simulink model "benchlink"  (R2024b)
settings: Solver=FixedStepDiscrete  StartTime=0.0  StopTime=0.005*16  RelTol=1e-3
model workspace (MAT data in the model file):
  socvcb : containers.Map (value not decoded)
values from neighbouring files (symbols this model uses):
  access = [32 0 4 36 32 0 4 36 32 0 4 36 ... (16 elements, 16x1)]    [all_variables.mat]
  qam_params =     [all_variables.mat]
undefined symbols (not defined in the file or in its folder): Add, j, QAM, rms, Shift
libraries: hdlsllib x53, simulink_need_slupdate x22, simulink x18, dspsigops x16, commdigbbndam3 x6, dsphdlmathfun2 x2, commchan3 x1, commrflib2 x1, dsphdlsigops2 x1, dspstat3 x1, dsphdlfiltering2 x1, simulink_extras x1
(part 4 of 5)

== system benchlink/HDL_64QAM/HDLRxIPCore/QAM Rx HDL/MF Filtering and Despreading/SymEVM ==
  chipValid : Inport
  chips : Inport  Port=2
  switchControl : Inport  Port=3
  " Integrate and Dump" : MATLAB Function  TreatAsAtomicUnit=on
  Add2 : Sum  Inputs=-+  OutDataTypeStr=fixdt(1,16,11)  SaturateOnIntegerOverflow=on
  Constant1 : Constant  Value=complex(0,0)  OutDataTypeStr=fixdt(1,32,15)  SampleTime=1/qam_params.chipRate
  Data Type Conversion3 : DataTypeConversion  OutDataTypeStr=fixdt(1,16,14)  RndMeth=Floor
  Delay{1..3,5..9,11..13,15,20..21} (14 alike) : Delay  DelayLength=1  InitialCondition=0  UseCircularBuffer=on
  Delay14 : Delay  DelayLength=9  InitialCondition=0  UseCircularBuffer=on
  Delay4 : Delay  Commented=on  DelayLength=1  InitialCondition=0  UseCircularBuffer=on
  Modulus : Subsystem
  Rectangular QAM Demodulator Baseband1 : commdigbbndam3/Rectangular QAM Demodulator Baseband  M=64  OutType=Integer  DecType=Hard decision  VarSource=Dialog  Variance=1  Dec=Gray  Mapping=[0:15]  PowType=Min. distance between symbols  MinDist=2  AvgPow=0.66  PeakPow=1  Ph=0  outDtype1=boolean  outDtype2=Inherit via internal rule  derotateFactorWordLen=16  derotateFactorDataTypeStr=Inherit: Same word length as input  derotateFactorLastDataTypeStr=Inherit: Same word length as input  denormFactorWordLen=16  denormFactorDataTypeStr=Inherit: Same word length as input  denormFactorLastDataTypeStr=Inherit: Same word length as input  prodOutWordLen=32  prodOutOverflowMode=Wrap  prodOutRoundingMode=Floor  prodOutOvFlMode=off  prodOutOvFlModeLastStrValue=off  sumWordLen=32
  Rectangular QAM Modulator Baseband1 : commdigbbndam3/Rectangular QAM Modulator Baseband  M=64  InType=Integer  Enc=Gray  Mapping=[0:15]  PowType=Min. distance between symbols  MinDist=2  AvgPow=.66  PeakPow=1.1  Ph=0  outDtype=Fixed-point  outWordLen=16  outUDDataType=sfix(16)  outFracLenMode=Best precision  outFracLen=15  outDataTypeStr=fixdt(1,16)  outLastDataTypeStr=fixdt(1,16)
  SEL2 : MultiPortSwitch  DataPortOrder=Zero-based contiguous  Inputs=2  DiagnosticForDefault=None  zeroidx=on  OutDataTypeStr=fixdt(1,32,15)  InputSameDT=off
  Shift Arithmetic1 : ArithShift  BinPtShiftNumber=-3  BitShiftDirection=Right
  Shift Arithmetic2 : ArithShift  BinPtShiftNumber=3  BitShiftDirection=Right
  Symbol Accum : Subsystem
  Unit Delay Enabled1 : simulink_need_slupdate/Unit Delay Enabled  vinit=0.0  tsamp=-1
  EVM : Outport  InitialOutput=0  VectorParamsAs1DForOutWhenUnconnected=off
  wires:
  chips/1 -> Delay13/1
  Delay21/1 -> Delay1/1
  Delay20/1 -> Data Type Conversion3/1
  " Integrate and Dump"/2(sumOut) -> Delay20/1
  " Integrate and Dump"/1(validOut) -> Delay21/1
  Delay13/1 -> " Integrate and Dump"/2(symbolIn)
  Symbol Accum/2(ValidOut) -> Unit Delay Enabled1/2
  Symbol Accum/1(Out) -> Unit Delay Enabled1/1
  Delay14/1 -> Symbol Accum/1(SwCtrl)
  Delay11/1 -> Delay12/1
  Data Type Conversion3/1 -> Shift Arithmetic2/1
  Modulus/1(dataOut) -> Delay15/1
  Unit Delay Enabled1/1 -> EVM/1
  Add2/1 -> Shift Arithmetic1/1  "e"
  Rectangular QAM Modulator Baseband1/1 -> Delay7/1
  Delay6/1 -> Rectangular QAM Demodulator Baseband1/1
  Delay12/1 -> Delay8/1
  Delay15/1 -> Symbol Accum/2(In)
  Delay9/1 -> Rectangular QAM Modulator Baseband1/1
  Rectangular QAM Demodulator Baseband1/1 -> Delay9/1
  Constant1/1 -> SEL2/2
  SEL2/1 -> Add2/1
  Delay1/1 -> Delay2/1
  Delay2/1 -> Delay5/1
  chipValid/1 -> Delay3/1
  Delay3/1 -> [chipValid], " Integrate and Dump"/1(dValid)
  [chipValid] -> Delay14/1
  Shift Arithmetic2/1 -> Delay6/1, Delay11/1
  Shift Arithmetic1/1 -> Modulus/1(dataIn)
  Delay8/1 -> Add2/2
  Delay7/1 -> SEL2/3
  Delay5/1 -> SEL2/1
  switchControl/1 -> Symbol Accum/3(switchControl)

== system benchlink/HDL_64QAM/HDLRxIPCore/QAM Rx HDL/Payload Delimiter/Normalized Modulus ==
  dataIn : Inport
  switchControl : Inport  Port=2
  Abs : Abs
  Abs1 : Abs
  Add : Sum  OutDataTypeStr=fixdt(0,8,8)  SaturateOnIntegerOverflow=on
  Add7 : Sum  SaturateOnIntegerOverflow=on
  Complex to Real-Imag2 : ComplexToRealImag
  Constant1 : Constant  Value=2^(-14)  OutDataTypeStr=fixdt(0,16,14)  SampleTime=-1
  Delay{1..9,15..16} (11 alike) : Delay  DelayLength=1  InitialCondition=0
  Delay10 : Delay  DelayLength=length(PreAmb)  InitialCondition=0
  Gain4 : Gain  Gain=0.4  OutDataTypeStr=fixdt(1,16,15)  SaturateOnIntegerOverflow=on
  KeepMax : MATLAB Function  TreatAsAtomicUnit=on
  KeepMaxSmallBurst : MATLAB Function  TreatAsAtomicUnit=on
  MinMax : MinMax  Inputs=2  SaturateOnIntegerOverflow=on
  MinMax1 : MinMax  Function=max  Inputs=2  SaturateOnIntegerOverflow=on
  Multiport Switch : MultiPortSwitch  Inputs=2  SaturateOnIntegerOverflow=off  InputSameDT=off
  Product : Product  SaturateOnIntegerOverflow=on
  Reciprocal : Product  Inputs=/  OutDataTypeStr=fixdt(0,8,1)  RndMeth=Zero  SaturateOnIntegerOverflow=on
  dataOut : Outport  VectorParamsAs1DForOutWhenUnconnected=off
  dataOutN : Outport  Port=2  VectorParamsAs1DForOutWhenUnconnected=off
  wires:
  dataIn/1 -> Complex to Real-Imag2/1
  Abs1/1 -> Delay1/1
  Abs/1 -> Delay4/1
  Gain4/1 -> Delay6/1
  MinMax1/1 -> Delay2/1  "|L|"
  MinMax/1 -> Delay7/1  "|Q|"
  Add7/1 -> Delay5/1
  Delay7/1 -> Gain4/1
  Delay2/1 -> Delay3/1
  Delay1/1 -> MinMax1/2, MinMax/2
  Delay4/1 -> MinMax1/1, MinMax/1
  Delay6/1 -> Add7/2
  Delay3/1 -> Add7/1
  Complex to Real-Imag2/2 -> Abs1/1  "Q"
  Complex to Real-Imag2/1 -> Abs/1  "I"
  Delay15/1 -> Add/1
  Add/1 -> Reciprocal/1
  Constant1/1 -> Add/2
  Product/1 -> Delay16/1
  KeepMax/1(out) -> Multiport Switch/2
  Delay16/1 -> dataOutN/1
  Delay8/1 -> Product/1, Delay9/1
  Delay9/1 -> dataOut/1
  Delay5/1 -> Delay10/1, KeepMaxSmallBurst/1(in), KeepMax/1(in)
  Delay10/1 -> Delay8/1
  Reciprocal/1 -> Product/2
  switchControl/1 -> Multiport Switch/1
  KeepMaxSmallBurst/1(out) -> Multiport Switch/3
  Multiport Switch/1 -> Delay15/1

== system benchlink/HDL_64QAM/HDLRxIPCore/QAM Rx HDL/Payload Delimiter/Peak Detector ==
  xCorr : Inport
  Threshold : Inport  Port=2
  Compare To Zero : simulink/Logic and Bit Operations/Compare To Zero  relop=>  OutDataTypeStr=boolean
  Compare To Zero1 : simulink/Logic and Bit Operations/Compare To Zero  relop=>  OutDataTypeStr=boolean
  Delay : Delay  DelayLength=1
  Delay1 : Delay
  Delay4 : Delay  DelayLength=1
  Logical Operator1 : Logic  AllPortsSameDT=off  OutDataTypeStr=boolean
  Logical Operator3 : Logic  AllPortsSameDT=off  OutDataTypeStr=boolean
  Subtract1 : Sum  Inputs=-+
  Subtract2 : Sum  Inputs=+-
  Out1 : Outport  VectorParamsAs1DForOutWhenUnconnected=off
  wires:
  Threshold/1 -> Delay4/1
  Delay/1 -> Subtract1/2, Subtract2/1
  Delay1/1 -> Subtract2/2
  xCorr/1 -> Delay1/1, Subtract1/1, Delay/1
  Delay4/1 -> Logical Operator3/1
  Subtract1/1 -> Compare To Zero/1
  Subtract2/1 -> Compare To Zero1/1
  Compare To Zero/1 -> Logical Operator1/1
  Compare To Zero1/1 -> Logical Operator1/2
  Logical Operator1/1 -> Logical Operator3/2
  Logical Operator3/1 -> Out1/1

== system benchlink/HDL_64QAM/HDLRxIPCore/QAM Rx HDL/Payload Delimiter/Preamble Matched Filter ==
  dataIn : Inport
  Add2 : Sum  SaturateOnIntegerOverflow=on
  Add3 : Sum  SaturateOnIntegerOverflow=on
  Complex to Real-Imag2 : ComplexToRealImag
  Delay{1,4..6} (4 alike) : Delay  DelayLength=1  InitialCondition=0
  Discrete FIR Filter1 : DiscreteFir  FilterStructure=Direct form transposed  Coefficients=sign(real(fliplr(PreAmb)))  CoefDataTypeStr=fixdt(1,2,0)  ProductDataTypeStr=fixdt(1,16,15)  AccumDataTypeStr=fixdt(1,24,15)  OutDataTypeStr=fixdt(1,24,15)  SaturateOnIntegerOverflow=on
  Discrete FIR Filter2 : DiscreteFir  FilterStructure=Direct form transposed  Coefficients=sign(imag(fliplr(PreAmb)))  CoefDataTypeStr=fixdt(1,2,0)  ProductDataTypeStr=fixdt(1,16,15)  AccumDataTypeStr=fixdt(1,24,15)  OutDataTypeStr=fixdt(1,24,15)  SaturateOnIntegerOverflow=on
  Gain : Gain  Gain=1/length(PreAmb)  OutDataTypeStr=fixdt(1,17,15)  SaturateOnIntegerOverflow=on
  Gain1 : Gain  Gain=1/length(PreAmb)  OutDataTypeStr=fixdt(1,17,15)  SaturateOnIntegerOverflow=on
  Real-Imag to Complex1 : RealImagToComplex
  dataOut : Outport  VectorParamsAs1DForOutWhenUnconnected=off
  wires:
  Delay1/1 -> Discrete FIR Filter2/1
  Delay4/1 -> Discrete FIR Filter1/1
  Add3/1 -> Delay1/1
  Add2/1 -> Delay4/1
  Complex to Real-Imag2/1 -> Add3/1, Add2/1
  Complex to Real-Imag2/2 -> Add2/2, Add3/2
  dataIn/1 -> Complex to Real-Imag2/1
  Delay5/1 -> Real-Imag to Complex1/1
  Delay6/1 -> Real-Imag to Complex1/2
  Gain/1 -> Delay5/1
  Discrete FIR Filter1/1 -> Gain/1
  Discrete FIR Filter2/1 -> Gain1/1
  Gain1/1 -> Delay6/1
  Real-Imag to Complex1/1 -> dataOut/1

== system benchlink/HDL_64QAM/HDLRxIPCore/QAM Rx HDL/Payload Delimiter/Rising Edge Detector ==
  In1 : Inport
  Compare To Constant7 : simulink/Logic and Bit Operations/Compare To Constant  relop===  const=1  OutDataTypeStr=boolean
  Data Type Conversion : DataTypeConversion  OutDataTypeStr=fixdt(1,2,0)  SaturateOnIntegerOverflow=off  RndMeth=Floor
  Data Type Conversion1 : DataTypeConversion  OutDataTypeStr=fixdt(1,2,0)  SaturateOnIntegerOverflow=off  RndMeth=Floor
  Data Type Conversion2 : DataTypeConversion  OutDataTypeStr=fixdt(1,2,0)  SaturateOnIntegerOverflow=off  RndMeth=Floor
  Delay1 : Delay  DelayLength=1  InitialCondition=0
  Subtract1 : Sum  Inputs=-+
  Out1 : Outport  VectorParamsAs1DForOutWhenUnconnected=off
  wires:
  In1/1 -> Data Type Conversion1/1, Delay1/1
  Delay1/1 -> Data Type Conversion/1
  Subtract1/1 -> Data Type Conversion2/1
  Data Type Conversion/1 -> Subtract1/1
  Data Type Conversion1/1 -> Subtract1/2
  Data Type Conversion2/1 -> Compare To Constant7/1
  Compare To Constant7/1 -> Out1/1

== system benchlink/HDL_64QAM/HDLRxIPCore/QAM Rx HDL/Payload Delimiter/frameIndexing ==
  rst : Inport
  switchControl : Inport  Port=2
  Frame Indexer1 : hdlsllib/Sources/HDL Counter  CountType=Count limited  CountInit=0  CountStep=1  CountMax=qam_params.packetSymLength*qam_params.spreadingFactor/4-1  CountFromType=Initial value  CountFrom=0  CountResetPort=on  CountLoadPort=off  CountEnbPort=off  CountDirPort=off  CountHitOutputPort=off  CountDataType=Unsigned  CountWordLen=32  CountFracLen=0  CountSampTime=1
  Frame Indexer2 : hdlsllib/Sources/HDL Counter  CountType=Free running  CountInit=0  CountStep=1  CountMax=qam_params.packetSymLength*qam_params.spreadingFactor-1  CountFromType=Initial value  CountFrom=0  CountResetPort=on  CountLoadPort=off  CountEnbPort=off  CountDirPort=off  CountHitOutputPort=off  CountDataType=Unsigned  CountWordLen=32  CountFracLen=0  CountSampTime=1
  Frame Indexer3 : hdlsllib/Sources/HDL Counter  CountType=Count limited  CountInit=0  CountStep=1  CountMax=qam_params.packetSymLengthBig*qam_params.spreadingFactor/8-1  CountFromType=Initial value  CountFrom=0  CountResetPort=on  CountLoadPort=off  CountEnbPort=off  CountDirPort=off  CountHitOutputPort=off  CountDataType=Unsigned  CountWordLen=32  CountFracLen=0  CountSampTime=1
  HDL Counter : hdlsllib/Sources/HDL Counter  CountType=Free running  CountInit=0  CountStep=1  CountMax=25  CountFromType=Initial value  CountFrom=0  CountResetPort=on  CountLoadPort=off  CountEnbPort=off  CountDirPort=off  CountHitOutputPort=off  CountDataType=Unsigned  CountWordLen=32  CountFracLen=0  CountSampTime=1
  Multiport Switch : MultiPortSwitch  Inputs=2  SaturateOnIntegerOverflow=off  InputSameDT=off
  Switch : Switch  Threshold=qam_params.packetSymLength*qam_params.spreadingFactor  SaturateOnIntegerOverflow=off  InputSameDT=off
  Switch1 : Switch  Threshold=qam_params.packetSymLengthBig*qam_params.spreadingFactor  SaturateOnIntegerOverflow=off  InputSameDT=off
  Out1 : Outport
  wires:
  rst/1 -> Frame Indexer1/1, HDL Counter/1, Frame Indexer2/1, Frame Indexer3/1
  HDL Counter/1 -> Switch/1, Switch/2
  switchControl/1 -> Multiport Switch/1
  Frame Indexer1/1 -> Switch/3
  Frame Indexer2/1 -> Switch1/1, Switch1/2
  Multiport Switch/1 -> Out1/1
  Switch1/1 -> Multiport Switch/3
  Frame Indexer3/1 -> Switch1/3
  Switch/1 -> Multiport Switch/2

== system benchlink/HDL_64QAM/HDLTxIPCore/QAMTxHDL/Async FIFO/Enabled Subsystem1 ==
  In1 : Inport
  hold : Inport  Port=2
  Memory : Memory  InheritSampleTime=on
  Switch1 : Switch  Criteria=u2 > Threshold  SaturateOnIntegerOverflow=off  InputSameDT=off
  access_per_burst : Outport
  wires:
  In1/1 -> Switch1/1
  Memory/1 -> Switch1/3
  Switch1/1 -> access_per_burst/1, Memory/1
  hold/1 -> Switch1/2

== system benchlink/HDL_64QAM/HDLTxIPCore/QAMTxHDL/Async FIFO/Enabled Wire ==
  In1 : Inport
  Enable : EnablePort
  rdyFromDown : Outport  InitialOutput=0  VectorParamsAs1DForOutWhenUnconnected=off
  wires:
  In1/1 -> rdyFromDown/1

== system benchlink/HDL_64QAM/HDLTxIPCore/QAMTxHDL/Subsystem2/Edge Detector ==
  In1 : Inport
  Delay : Delay  DelayLength=1
  XOR : Logic  Operator=XOR  IconShape=distinctive  AllPortsSameDT=off  OutDataTypeStr=boolean
  Out1 : Outport  VectorParamsAs1DForOutWhenUnconnected=off
  wires:
  In1/1 -> XOR/1, Delay/1
  Delay/1 -> XOR/2
  XOR/1 -> Out1/1

== system benchlink/HDL_64QAM/HDLRxIPCore/QAM Rx HDL/DA CFC_Avg/Frequency Offset Estimation/Autocorrelation Estimate ==
  dataIn : Inport
  Add : Sum  OutDataTypeStr=fixdt(1,64,46)  AccumDataTypeStr=fixdt(1,64,46)
  Complex to Real-Imag : ComplexToRealImag
  Conjugate : Math  Operator=conj  SignedPower=on  RndMeth=Zero
  Delay : Delay  DelayLength=qam_params.spreadingFactor
  Delay{1..7} (7 alike) : Delay  DelayLength=1  InitialCondition=0  UseCircularBuffer=on
  Moving_Average : Subsystem
  Product : Product  OutDataTypeStr=fixdt(1,32,18)  RndMeth=Round
  Product1 : Product  OutDataTypeStr=fixdt(1,64,46)
  Product2 : Product  OutDataTypeStr=fixdt(1,64,4)
  corr : Outport  VectorParamsAs1DForOutWhenUnconnected=off
  corrAbs : Outport  Port=2  VectorParamsAs1DForOutWhenUnconnected=off
  wires:
  Product/1 -> Delay5/1
  Delay3/1 -> Product/2
  Delay1/1 -> Product/1
  dataIn/1 -> Delay1/1, Delay/1
  Conjugate/1 -> Delay3/1
  Moving_Average/1(dataOut) -> Delay2/1
  Product1/1 -> Delay6/1
  Product2/1 -> Delay4/1
  Add/1 -> corrAbs/1
  Complex to Real-Imag/1 -> Product1/1, Product1/2
  Complex to Real-Imag/2 -> Product2/2, Product2/1
  Delay4/1 -> Add/2
  Delay6/1 -> Add/1
  Delay/1 -> Conjugate/1
  Delay2/1 -> Delay7/1, Complex to Real-Imag/1
  Delay5/1 -> Moving_Average/1(dataIn)
  Delay7/1 -> corr/1

== system benchlink/HDL_64QAM/HDLRxIPCore/QAM Rx HDL/DA CFC_Avg/Frequency Offset Estimation/Latch ==
  S : Inport
  R : Inport  Port=2
  Delay2 : Delay  DelayLength=1  InitialCondition=0
  Logical Operator : Logic  Operator=OR  AllPortsSameDT=off  OutDataTypeStr=boolean
  Logical Operator1 : Logic  AllPortsSameDT=off  OutDataTypeStr=boolean
  Logical Operator2 : Logic  Operator=NOT  AllPortsSameDT=off  OutDataTypeStr=boolean
  Q : Outport  VectorParamsAs1DForOutWhenUnconnected=off
  wires:
  R/1 -> Logical Operator2/1
  S/1 -> Logical Operator/1
  Logical Operator/1 -> Delay2/1
  Logical Operator1/1 -> Logical Operator/2
  Logical Operator2/1 -> Logical Operator1/1
  Delay2/1 -> Q/1, Logical Operator1/2

== system benchlink/HDL_64QAM/HDLRxIPCore/QAM Rx HDL/DA CFC_Avg/Frequency Offset Estimation/Moving_Average ==
  dataIn : Inport
  Add : Sum  Inputs=-+  AccumDataTypeStr=fixdt(1,32,18)
  Add1 : Sum  OutDataTypeStr=fixdt(1,32,18)  AccumDataTypeStr=fixdt(1,32,18)
  Delay : Delay  DelayLength=qam_params.spreadingFactor-1
  Delay10 : Delay  DelayLength=1  InitialCondition=0  UseCircularBuffer=on
  Delay4 : Delay  DelayLength=1  InitialCondition=0  UseCircularBuffer=on
  Gain : Gain  Gain=1/(qam_params.longTrainingChipLength/4)  OutDataTypeStr=fixdt(1,32,23)
  dataOut : Outport  VectorParamsAs1DForOutWhenUnconnected=off
  wires:
  Add/1 -> Delay10/1
  dataIn/1 -> Delay/1, Add/2
  Delay10/1 -> Add1/2
  Add1/1 -> Gain/1, Delay4/1
  Delay/1 -> Add/1
  Delay4/1 -> Add1/1
  Gain/1 -> dataOut/1

== system benchlink/HDL_64QAM/HDLRxIPCore/QAM Rx HDL/DA CFC_Avg/Frequency Offset Estimation/Peak Detector ==
  xCorr : Inport
  Threshold : Inport  Port=2
  Compare To Zero : simulink/Logic and Bit Operations/Compare To Zero  relop=>  OutDataTypeStr=boolean
  Compare To Zero1 : simulink/Logic and Bit Operations/Compare To Zero  relop=>  OutDataTypeStr=boolean
  Delay : Delay  DelayLength=1
  Delay1 : Delay
  Delay4 : Delay  DelayLength=1
  Logical Operator1 : Logic  AllPortsSameDT=off  OutDataTypeStr=boolean
  Logical Operator3 : Logic  AllPortsSameDT=off  OutDataTypeStr=boolean
  Subtract1 : Sum  Inputs=-+
  Subtract2 : Sum  Inputs=+-
  Out1 : Outport  VectorParamsAs1DForOutWhenUnconnected=off
  wires:
  Threshold/1 -> Delay4/1
  Delay/1 -> Subtract1/2, Subtract2/1
  Delay1/1 -> Subtract2/2
  xCorr/1 -> Delay1/1, Subtract1/1, Delay/1
  Delay4/1 -> Logical Operator3/1
  Subtract1/1 -> Compare To Zero/1
  Subtract2/1 -> Compare To Zero1/1
  Compare To Zero/1 -> Logical Operator1/1
  Compare To Zero1/1 -> Logical Operator1/2
  Logical Operator1/1 -> Logical Operator3/2
  Logical Operator3/1 -> Out1/1

== system benchlink/HDL_64QAM/HDLRxIPCore/QAM Rx HDL/DA CFC_Avg/Frequency Offset Estimation/Rising Edge Detector ==
  In1 : Inport
  Compare To Constant7 : simulink/Logic and Bit Operations/Compare To Constant  relop===  const=1  OutDataTypeStr=boolean
  Data Type Conversion : DataTypeConversion  OutDataTypeStr=fixdt(1,2,0)  SaturateOnIntegerOverflow=off  RndMeth=Floor
  Data Type Conversion1 : DataTypeConversion  OutDataTypeStr=fixdt(1,2,0)  SaturateOnIntegerOverflow=off  RndMeth=Floor
  Data Type Conversion2 : DataTypeConversion  OutDataTypeStr=fixdt(1,2,0)  SaturateOnIntegerOverflow=off  RndMeth=Floor
  Delay1 : Delay  DelayLength=1  InitialCondition=0
  Subtract1 : Sum  Inputs=-+
  Out1 : Outport  VectorParamsAs1DForOutWhenUnconnected=off
  wires:
  In1/1 -> Data Type Conversion1/1, Delay1/1
  Delay1/1 -> Data Type Conversion/1
  Subtract1/1 -> Data Type Conversion2/1
  Data Type Conversion/1 -> Subtract1/1
  Data Type Conversion1/1 -> Subtract1/2
  Data Type Conversion2/1 -> Compare To Constant7/1
  Compare To Constant7/1 -> Out1/1

== system benchlink/HDL_64QAM/HDLRxIPCore/QAM Rx HDL/DA CFC_Avg/Frequency Offset Estimation/Variance Estimate ==
  dataIn : Inport
  Complex to Real-Imag1 : ComplexToRealImag  Output=Real
  Conjugate : Math  Operator=conj  SignedPower=on  RndMeth=Zero
  Delay{1..3,5..7} (6 alike) : Delay  DelayLength=1  InitialCondition=0  UseCircularBuffer=on
  Moving_Average : Subsystem
  Product : Product  OutDataTypeStr=fixdt(1,32,18)  RndMeth=Round
  Product1 : Product  OutDataTypeStr=fixdt(1,64,46)
  var : Outport  VectorParamsAs1DForOutWhenUnconnected=off
  varAbs : Outport  Port=2  VectorParamsAs1DForOutWhenUnconnected=off
  wires:
  Product/1 -> Complex to Real-Imag1/1
  Delay3/1 -> Product/2
  Delay1/1 -> Product/1
  Conjugate/1 -> Delay3/1
  Moving_Average/1(dataOut) -> Delay2/1
  Product1/1 -> Delay6/1
  Delay6/1 -> varAbs/1
  dataIn/1 -> Conjugate/1, Delay1/1
  Delay5/1 -> Moving_Average/1(dataIn)
  Complex to Real-Imag1/1 -> Delay5/1
  Delay7/1 -> var/1
  Delay2/1 -> Delay7/1, Product1/1, Product1/2

== system benchlink/HDL_64QAM/HDLRxIPCore/QAM Rx HDL/Enabled AGC1/Energy Detector/Latch1 ==
  S : Inport
  R : Inport  Port=2
  Delay2 : Delay  DelayLength=1  InitialCondition=0
  Logical Operator : Logic  Operator=OR  AllPortsSameDT=off  OutDataTypeStr=boolean
  Logical Operator1 : Logic  AllPortsSameDT=off  OutDataTypeStr=boolean
  Logical Operator2 : Logic  Operator=NOT  AllPortsSameDT=off  OutDataTypeStr=boolean
  Q : Outport  VectorParamsAs1DForOutWhenUnconnected=off
  wires:
  R/1 -> Logical Operator2/1
  S/1 -> Logical Operator/1
  Logical Operator/1 -> Delay2/1
  Logical Operator1/1 -> Logical Operator/2
  Logical Operator2/1 -> Logical Operator1/1
  Delay2/1 -> Q/1, Logical Operator1/2

== system benchlink/HDL_64QAM/HDLRxIPCore/QAM Rx HDL/Enabled AGC1/Energy Detector/Variance Estimate ==
  dataIn : Inport
  Complex to Real-Imag1 : ComplexToRealImag  Output=Real
  Conjugate : Math  Operator=conj  SignedPower=on  RndMeth=Zero
  Delay{1..3,5..7} (6 alike) : Delay  DelayLength=1  InitialCondition=0  UseCircularBuffer=on
  Moving_Average : Subsystem
  Product : Product  OutDataTypeStr=fixdt(1,32,18)  RndMeth=Round
  Product1 : Product  OutDataTypeStr=fixdt(1,64,46)
  var : Outport  VectorParamsAs1DForOutWhenUnconnected=off
  varAbs : Outport  Port=2  VectorParamsAs1DForOutWhenUnconnected=off
  wires:
  Product/1 -> Complex to Real-Imag1/1
  Delay3/1 -> Product/2
  Delay1/1 -> Product/1
  Conjugate/1 -> Delay3/1
  Moving_Average/1(dataOut) -> Delay2/1
  Product1/1 -> Delay6/1
  Delay6/1 -> varAbs/1
  dataIn/1 -> Conjugate/1, Delay1/1
  Delay5/1 -> Moving_Average/1(dataIn)
  Complex to Real-Imag1/1 -> Delay5/1
  Delay7/1 -> var/1
  Delay2/1 -> Delay7/1, Product1/1, Product1/2

== system benchlink/HDL_64QAM/HDLRxIPCore/QAM Rx HDL/Enabled AGC1/Energy Detector/Variance Estimate2 ==
  dataIn : Inport
  Complex to Real-Imag1 : ComplexToRealImag  Output=Real
  Conjugate : Math  Operator=conj  SignedPower=on  RndMeth=Zero
  Delay{1..3,5..7} (6 alike) : Delay  DelayLength=1  InitialCondition=0  UseCircularBuffer=on
  Moving_Average : Subsystem
  Product : Product  OutDataTypeStr=fixdt(1,32,18)  RndMeth=Round
  Product1 : Product  OutDataTypeStr=fixdt(1,64,46)
  var : Outport  VectorParamsAs1DForOutWhenUnconnected=off
  varAbs : Outport  Port=2  VectorParamsAs1DForOutWhenUnconnected=off
  wires:
  Product/1 -> Complex to Real-Imag1/1
  Delay3/1 -> Product/2
  Delay1/1 -> Product/1
  Conjugate/1 -> Delay3/1
  Moving_Average/1(dataOut) -> Delay2/1
  Product1/1 -> Delay6/1
  Delay6/1 -> varAbs/1
  dataIn/1 -> Conjugate/1, Delay1/1
  Delay5/1 -> Moving_Average/1(dataIn)
  Complex to Real-Imag1/1 -> Delay5/1
  Delay7/1 -> var/1
  Delay2/1 -> Delay7/1, Product1/1, Product1/2

== system benchlink/HDL_64QAM/HDLRxIPCore/QAM Rx HDL/Enabled AGC2/Energy Detector/Latch1 ==
  S : Inport
  R : Inport  Port=2
  Delay2 : Delay  DelayLength=1  InitialCondition=0
  Logical Operator : Logic  Operator=OR  AllPortsSameDT=off  OutDataTypeStr=boolean
  Logical Operator1 : Logic  AllPortsSameDT=off  OutDataTypeStr=boolean
  Logical Operator2 : Logic  Operator=NOT  AllPortsSameDT=off  OutDataTypeStr=boolean
  Q : Outport  VectorParamsAs1DForOutWhenUnconnected=off
  wires:
  R/1 -> Logical Operator2/1
  S/1 -> Logical Operator/1
  Logical Operator/1 -> Delay2/1
  Logical Operator1/1 -> Logical Operator/2
  Logical Operator2/1 -> Logical Operator1/1
  Delay2/1 -> Q/1, Logical Operator1/2

== system benchlink/HDL_64QAM/HDLRxIPCore/QAM Rx HDL/Enabled AGC2/Energy Detector/Variance Estimate ==
  dataIn : Inport
  Complex to Real-Imag1 : ComplexToRealImag  Output=Real
  Conjugate : Math  Operator=conj  SignedPower=on  RndMeth=Zero
  Delay{1..3,5..7} (6 alike) : Delay  DelayLength=1  InitialCondition=0  UseCircularBuffer=on
  Moving_Average : Subsystem
  Product : Product  OutDataTypeStr=fixdt(1,32,18)  RndMeth=Round
  Product1 : Product  OutDataTypeStr=fixdt(1,64,46)
  var : Outport  VectorParamsAs1DForOutWhenUnconnected=off
  varAbs : Outport  Port=2  VectorParamsAs1DForOutWhenUnconnected=off
  wires:
  Product/1 -> Complex to Real-Imag1/1
  Delay3/1 -> Product/2
  Delay1/1 -> Product/1
  Conjugate/1 -> Delay3/1
  Moving_Average/1(dataOut) -> Delay2/1
  Product1/1 -> Delay6/1
  Delay6/1 -> varAbs/1
  dataIn/1 -> Conjugate/1, Delay1/1
  Delay5/1 -> Moving_Average/1(dataIn)
  Complex to Real-Imag1/1 -> Delay5/1
  Delay7/1 -> var/1
  Delay2/1 -> Delay7/1, Product1/1, Product1/2

== system benchlink/HDL_64QAM/HDLRxIPCore/QAM Rx HDL/Enabled AGC2/Energy Detector/Variance Estimate2 ==
  dataIn : Inport
  Complex to Real-Imag1 : ComplexToRealImag  Output=Real
  Conjugate : Math  Operator=conj  SignedPower=on  RndMeth=Zero
  Delay{1..3,5..7} (6 alike) : Delay  DelayLength=1  InitialCondition=0  UseCircularBuffer=on
  Moving_Average : Subsystem
  Product : Product  OutDataTypeStr=fixdt(1,32,18)  RndMeth=Round
  Product1 : Product  OutDataTypeStr=fixdt(1,64,46)
  var : Outport  VectorParamsAs1DForOutWhenUnconnected=off
  varAbs : Outport  Port=2  VectorParamsAs1DForOutWhenUnconnected=off
  wires:
  Product/1 -> Complex to Real-Imag1/1
  Delay3/1 -> Product/2
  Delay1/1 -> Product/1
  Conjugate/1 -> Delay3/1
  Moving_Average/1(dataOut) -> Delay2/1
  Product1/1 -> Delay6/1
  Delay6/1 -> varAbs/1
  dataIn/1 -> Conjugate/1, Delay1/1
  Delay5/1 -> Moving_Average/1(dataIn)
  Complex to Real-Imag1/1 -> Delay5/1
  Delay7/1 -> var/1
  Delay2/1 -> Delay7/1, Product1/1, Product1/2

== system benchlink/HDL_64QAM/HDLRxIPCore/QAM Rx HDL/Enabled AGC2/signal power1/Rising Edge Detector ==
  In1 : Inport
  Compare To Constant7 : simulink/Logic and Bit Operations/Compare To Constant  relop===  const=1  OutDataTypeStr=boolean
  Data Type Conversion : DataTypeConversion  OutDataTypeStr=fixdt(1,2,0)  SaturateOnIntegerOverflow=off  RndMeth=Floor
  Data Type Conversion1 : DataTypeConversion  OutDataTypeStr=fixdt(1,2,0)  SaturateOnIntegerOverflow=off  RndMeth=Floor
  Data Type Conversion2 : DataTypeConversion  OutDataTypeStr=fixdt(1,2,0)  SaturateOnIntegerOverflow=off  RndMeth=Floor
  Delay1 : Delay  DelayLength=1  InitialCondition=0
  Subtract1 : Sum  Inputs=-+
  Out1 : Outport  VectorParamsAs1DForOutWhenUnconnected=off
  wires:
  In1/1 -> Data Type Conversion1/1, Delay1/1
  Delay1/1 -> Data Type Conversion/1
  Subtract1/1 -> Data Type Conversion2/1
  Data Type Conversion/1 -> Subtract1/1
  Data Type Conversion1/1 -> Subtract1/2
  Data Type Conversion2/1 -> Compare To Constant7/1
  Compare To Constant7/1 -> Out1/1

== system benchlink/HDL_64QAM/HDLRxIPCore/QAM Rx HDL/Enabled AGC2/signal power1/power1 ==
  x : Inport
  Complex to Real-Imag : ComplexToRealImag
  Delay : Delay  InitialCondition=0
  Delay1 : Delay  InitialCondition=0
  Delay3 : Delay  InitialCondition=0
  Product3 : Product  OutDataTypeStr=fixdt(1,16,15)  SaturateOnIntegerOverflow=on
  Product4 : Product  OutDataTypeStr=fixdt(1,16,15)  SaturateOnIntegerOverflow=on
  Sum1 : Sum  OutDataTypeStr=fixdt(1,16,14)  AccumDataTypeStr=fixdt(1,16,15)  SaturateOnIntegerOverflow=on
  Out1 : Outport  VectorParamsAs1DForOutWhenUnconnected=off
  wires:
  Product3/1 -> Delay/1
  Complex to Real-Imag/1 -> Product3/2, Product3/1
  Complex to Real-Imag/2 -> Product4/1, Product4/2
  Product4/1 -> Delay1/1
  Sum1/1 -> Delay3/1
  Delay/1 -> Sum1/1
  Delay1/1 -> Sum1/2
  x/1 -> Complex to Real-Imag/1
  Delay3/1 -> Out1/1

== system benchlink/HDL_64QAM/HDLRxIPCore/QAM Rx HDL/MF Filtering and Despreading/BER/BER Avg ==
  codeVec : Inport
  enable : Inport  Port=2
  Delay{1..11,16} (12 alike) : Delay  DelayLength=1  InitialCondition=0
  Gain : Gain  Gain=1/8  OutDataTypeStr=fixdt(0,16,9)  SaturateOnIntegerOverflow=on
  MATLAB Function1 : MATLAB Function  TreatAsAtomicUnit=on
  MATLAB Function2 : MATLAB Function  Commented=on  TreatAsAtomicUnit=on
  Product : Product  OutDataTypeStr=fixdt(0,16,9)  SaturateOnIntegerOverflow=on
  Reciprocal : Product  Inputs=/  OutDataTypeStr=fixdt(0,8,7)  RndMeth=Zero  SaturateOnIntegerOverflow=on
  Switch : Switch  Criteria=u2 ~= 0  SaturateOnIntegerOverflow=off  InputSameDT=off
  avgVecOut : Outport  VectorParamsAs1DForOutWhenUnconnected=off
  wires:
  codeVec/1 -> Delay10/1
  Delay16/1 -> avgVecOut/1
  enable/1 -> Delay11/1
  Delay1/1 -> Delay4/1
  Switch/1 -> Delay16/1
  Gain/1 -> Delay7/1
  Delay7/1 -> Switch/1
  Delay8/1 -> Switch/2
  Product/1 -> Delay9/1
  Delay3/1 -> Reciprocal/1
  Reciprocal/1 -> Delay6/1
  Delay2/1 -> Delay5/1
  MATLAB Function1/1(BERSumOut) -> Delay1/1
  MATLAB Function1/2(vecFullOut) -> Delay2/1
  MATLAB Function1/3(countOut) -> Delay3/1
  Delay4/1 -> Product/1, Gain/1
  Delay5/1 -> Delay8/1
  Delay6/1 -> Product/2
  Delay9/1 -> Switch/3
  Delay10/1 -> MATLAB Function1/1(BERIn)
  Delay11/1 -> MATLAB Function1/2(enable)

== system benchlink/HDL_64QAM/HDLRxIPCore/QAM Rx HDL/MF Filtering and Despreading/BER/Symbol Accum1 ==
  SwCtrl : Inport
  In : Inport  Port=2
  Accum Scale : Gain  Gain=100/qam_params.bitsPerSymbol/qam_params.longTrainingChipLength  OutDataTypeStr=fixdt(0,16,9)  SaturateOnIntegerOverflow=on
  Add2 : Sum  OutDataTypeStr=uint16  SaturateOnIntegerOverflow=on
  Constant1 : Constant  Value=0  OutDataTypeStr=uint16  SampleTime=1/qam_params.chipRate
  Delay{1..3,14} (4 alike) : Delay  DelayLength=1  InitialCondition=0
  Enabled Wire : Subsystem  TreatAsAtomicUnit=on
      settings: RTWSystemCode=Nonreusable function
  Falling Edge Detector : Subsystem
  SEL2 : MultiPortSwitch  DataPortOrder=Zero-based contiguous  Inputs=2  DiagnosticForDefault=None  zeroidx=on  OutDataTypeStr=uint16  InputSameDT=off
  Unit Delay1 : UnitDelay  InitialCondition=0+0j  SampleTime=-1  HasFrameUpgradeWarning=on
  Out : Outport  VectorParamsAs1DForOutWhenUnconnected=off
  ValidOut : Outport  Port=2  VectorParamsAs1DForOutWhenUnconnected=off
  wires:
  Unit Delay1/1 -> SEL2/3, Accum Scale/1
  In/1 -> Delay2/1
  Add2/1 -> Unit Delay1/1
  SEL2/1 -> Add2/1
  SwCtrl/1 -> Delay14/1
  Accum Scale/1 -> Enabled Wire/1(In1)
  Enabled Wire/1(Out1) -> Delay1/1
  Constant1/1 -> SEL2/2
  Delay14/1 -> Falling Edge Detector/1(In1), SEL2/1
  Delay2/1 -> Add2/2
  Delay1/1 -> Out/1
  Falling Edge Detector/1(Out1) -> Delay3/1, Enabled Wire/Enable
  Delay3/1 -> ValidOut/1

== system benchlink/HDL_64QAM/HDLRxIPCore/QAM Rx HDL/MF Filtering and Despreading/Channel Estimation/Enabled Wire ==
  In1 : Inport
  Enable : EnablePort
  Out1 : Outport  InitialOutput=0  VectorParamsAs1DForOutWhenUnconnected=off
  wires:
  In1/1 -> Out1/1

== system benchlink/HDL_64QAM/HDLRxIPCore/QAM Rx HDL/MF Filtering and Despreading/Channel Estimation/Enabled Wire1 ==
  In1 : Inport
  Enable : EnablePort
  Out1 : Outport  InitialOutput=0  VectorParamsAs1DForOutWhenUnconnected=off
  wires:
  In1/1 -> Out1/1

== system benchlink/HDL_64QAM/HDLRxIPCore/QAM Rx HDL/MF Filtering and Despreading/Channel Estimation/Falling Edge Detector ==
  In1 : Inport
  Compare To Constant7 : simulink/Logic and Bit Operations/Compare To Constant  relop===  const=-1  OutDataTypeStr=boolean
  Data Type Conversion : DataTypeConversion  OutDataTypeStr=fixdt(1,2,0)  SaturateOnIntegerOverflow=off  RndMeth=Floor
  Data Type Conversion1 : DataTypeConversion  OutDataTypeStr=fixdt(1,2,0)  SaturateOnIntegerOverflow=off  RndMeth=Floor
  Data Type Conversion2 : DataTypeConversion  OutDataTypeStr=fixdt(1,2,0)  SaturateOnIntegerOverflow=off  RndMeth=Floor
  Delay1 : Delay  DelayLength=1  InitialCondition=0
  Subtract1 : Sum  Inputs=-+
  Out1 : Outport  VectorParamsAs1DForOutWhenUnconnected=off
  wires:
  In1/1 -> Data Type Conversion1/1, Delay1/1
  Delay1/1 -> Data Type Conversion/1
  Subtract1/1 -> Data Type Conversion2/1
  Data Type Conversion/1 -> Subtract1/1
  Data Type Conversion1/1 -> Subtract1/2
  Data Type Conversion2/1 -> Compare To Constant7/1
  Compare To Constant7/1 -> Out1/1

== system benchlink/HDL_64QAM/HDLRxIPCore/QAM Rx HDL/MF Filtering and Despreading/Desired Symbol Source/Rising Edge Detector ==
  In1 : Inport
  Compare To Constant7 : simulink/Logic and Bit Operations/Compare To Constant  relop===  const=1  OutDataTypeStr=boolean
  Data Type Conversion : DataTypeConversion  OutDataTypeStr=fixdt(1,2,0)  SaturateOnIntegerOverflow=off  RndMeth=Floor
  Data Type Conversion1 : DataTypeConversion  OutDataTypeStr=fixdt(1,2,0)  SaturateOnIntegerOverflow=off  RndMeth=Floor
  Data Type Conversion2 : DataTypeConversion  OutDataTypeStr=fixdt(1,2,0)  SaturateOnIntegerOverflow=off  RndMeth=Floor
  Delay1 : Delay  DelayLength=1  InitialCondition=0
  Subtract1 : Sum  Inputs=-+
  Out1 : Outport  VectorParamsAs1DForOutWhenUnconnected=off
  wires:
  In1/1 -> Data Type Conversion1/1, Delay1/1
  Delay1/1 -> Data Type Conversion/1
  Subtract1/1 -> Data Type Conversion2/1
  Data Type Conversion/1 -> Subtract1/1
  Data Type Conversion1/1 -> Subtract1/2
  Data Type Conversion2/1 -> Compare To Constant7/1
  Compare To Constant7/1 -> Out1/1

== system benchlink/HDL_64QAM/HDLRxIPCore/QAM Rx HDL/MF Filtering and Despreading/SymEVM/Modulus ==
  dataIn : Inport
  Abs : Abs  SaturateOnIntegerOverflow=off
  Abs1 : Abs  SaturateOnIntegerOverflow=off
  Add7 : Sum
  Complex to Real-Imag2 : ComplexToRealImag
  Delay{1..7} (7 alike) : Delay  DelayLength=1  InitialCondition=0
  Gain4 : Gain  Gain=0.4  OutDataTypeStr=fixdt(1,16,15)
  MinMax : MinMax  Inputs=2
  MinMax1 : MinMax  Function=max  Inputs=2
  dataOut : Outport  VectorParamsAs1DForOutWhenUnconnected=off
  wires:
  dataIn/1 -> Complex to Real-Imag2/1
  Abs1/1 -> Delay1/1
  Abs/1 -> Delay4/1
  Gain4/1 -> Delay6/1
  MinMax1/1 -> Delay2/1  "|L|"
  MinMax/1 -> Delay7/1  "|Q|"
  Add7/1 -> Delay5/1
  Delay7/1 -> Gain4/1
  Delay2/1 -> Delay3/1
  Delay1/1 -> MinMax1/2, MinMax/2
  Delay4/1 -> MinMax1/1, MinMax/1
  Delay6/1 -> Add7/2
  Delay5/1 -> dataOut/1
  Delay3/1 -> Add7/1
  Complex to Real-Imag2/2 -> Abs1/1  "Q"
  Complex to Real-Imag2/1 -> Abs/1  "I"

== system benchlink/HDL_64QAM/HDLRxIPCore/QAM Rx HDL/MF Filtering and Despreading/SymEVM/Symbol Accum ==
  SwCtrl : Inport
  In : Inport  Port=2
  switchControl : Inport  Port=3
  Accum Scale : Gain  Gain=100/qam_params.packetSymLength/sqrt(0.6556)  OutDataTypeStr=fixdt(1,32,15)  SaturateOnIntegerOverflow=on
  Accum Scale1 : Gain  Gain=100/qam_params.packetSymLengthBig/sqrt(0.6556)  OutDataTypeStr=fixdt(1,32,15)  SaturateOnIntegerOverflow=on
  Add2 : Sum  OutDataTypeStr=fixdt(1,32,15)  SaturateOnIntegerOverflow=on
  Constant1 : Constant  Value=0  OutDataTypeStr=fixdt(1,32,15)  SampleTime=1/qam_params.chipRate
  Delay{1..3,14} (4 alike) : Delay  DelayLength=1  InitialCondition=0
  Enabled Wire : Subsystem  TreatAsAtomicUnit=on
      settings: RTWSystemCode=Nonreusable function
  Falling Edge Detector : Subsystem
  Multiport Switch : MultiPortSwitch  Inputs=2  SaturateOnIntegerOverflow=off  InputSameDT=off
  SEL2 : MultiPortSwitch  DataPortOrder=Zero-based contiguous  Inputs=2  DiagnosticForDefault=None  zeroidx=on  OutDataTypeStr=fixdt(1,32,15)  InputSameDT=off
  Unit Delay1 : UnitDelay  InitialCondition=0+0j  SampleTime=-1  HasFrameUpgradeWarning=on
  Out : Outport  VectorParamsAs1DForOutWhenUnconnected=off
  ValidOut : Outport  Port=2  VectorParamsAs1DForOutWhenUnconnected=off
  wires:
  Unit Delay1/1 -> Accum Scale1/1, SEL2/3, Accum Scale/1
  In/1 -> Delay2/1
  Add2/1 -> Unit Delay1/1
  SEL2/1 -> Add2/1
  SwCtrl/1 -> Delay14/1
  Accum Scale/1 -> Multiport Switch/2
  Enabled Wire/1(Out1) -> Delay1/1
  Constant1/1 -> SEL2/2
  Delay14/1 -> Falling Edge Detector/1(In1), SEL2/1
  Delay2/1 -> Add2/2
  Delay1/1 -> Out/1
  Falling Edge Detector/1(Out1) -> Delay3/1, Enabled Wire/Enable
  Delay3/1 -> ValidOut/1
  switchControl/1 -> Multiport Switch/1
  Accum Scale1/1 -> Multiport Switch/3
  Multiport Switch/1 -> Enabled Wire/1(In1)

== system benchlink/HDL_64QAM/HDLRxIPCore/QAM Rx HDL/DA CFC_Avg/Frequency Offset Estimation/Autocorrelation Estimate/Moving_Average ==
  dataIn : Inport
  Add : Sum  Inputs=-+  AccumDataTypeStr=fixdt(1,32,18)
  Add1 : Sum  OutDataTypeStr=fixdt(1,32,18)  AccumDataTypeStr=fixdt(1,32,18)
  Delay : Delay  DelayLength=qam_params.trainingLength-qam_params.spreadingFactor
  Delay10 : Delay  DelayLength=1  InitialCondition=0  UseCircularBuffer=on
  Delay4 : Delay  DelayLength=1  InitialCondition=0  UseCircularBuffer=on
  Gain : Gain  Gain=1/(qam_params.longTrainingChipLength/4)  OutDataTypeStr=fixdt(1,32,23)
  dataOut : Outport  VectorParamsAs1DForOutWhenUnconnected=off
  wires:
  Add/1 -> Delay10/1
  dataIn/1 -> Delay/1, Add/2
  Delay10/1 -> Add1/2
  Add1/1 -> Gain/1, Delay4/1
  Delay/1 -> Add/1
  Delay4/1 -> Add1/1
  Gain/1 -> dataOut/1

== system benchlink/HDL_64QAM/HDLRxIPCore/QAM Rx HDL/DA CFC_Avg/Frequency Offset Estimation/Variance Estimate/Moving_Average ==
  dataIn : Inport
  Add : Sum  Inputs=-+  AccumDataTypeStr=fixdt(1,32,18)
  Add1 : Sum  OutDataTypeStr=fixdt(1,32,18)  AccumDataTypeStr=fixdt(1,32,18)
  Delay : Delay  DelayLength=qam_params.trainingLength-qam_params.spreadingFactor
  Delay10 : Delay  DelayLength=1  InitialCondition=0  UseCircularBuffer=on
  Delay4 : Delay  DelayLength=1  InitialCondition=0  UseCircularBuffer=on
  Gain : Gain  Gain=1/(qam_params.longTrainingChipLength/4)  OutDataTypeStr=fixdt(1,32,23)
  dataOut : Outport  VectorParamsAs1DForOutWhenUnconnected=off
  wires:
  Add/1 -> Delay10/1
  dataIn/1 -> Delay/1, Add/2
  Delay10/1 -> Add1/2
  Add1/1 -> Gain/1, Delay4/1
  Delay/1 -> Add/1
  Delay4/1 -> Add1/1
  Gain/1 -> dataOut/1

== system benchlink/HDL_64QAM/HDLRxIPCore/QAM Rx HDL/Enabled AGC1/Energy Detector/Variance Estimate/Moving_Average ==
  dataIn : Inport
  Add : Sum  Inputs=-+  AccumDataTypeStr=fixdt(1,32,18)
  Add1 : Sum  OutDataTypeStr=fixdt(1,32,18)  AccumDataTypeStr=fixdt(1,32,18)
  Delay : Delay  DelayLength=qam_params.golayLength*qam_params.Upsampling*3
  Delay10 : Delay  DelayLength=1  InitialCondition=0  UseCircularBuffer=on
  Delay4 : Delay  DelayLength=1  InitialCondition=0  UseCircularBuffer=on
  Gain : Gain  Gain=1/(qam_params.longTrainingChipLength/4)  OutDataTypeStr=fixdt(1,32,23)
  dataOut : Outport  VectorParamsAs1DForOutWhenUnconnected=off
  wires:
  Add/1 -> Delay10/1
  dataIn/1 -> Delay/1, Add/2
  Delay10/1 -> Add1/2
  Add1/1 -> Gain/1, Delay4/1
  Delay/1 -> Add/1
  Delay4/1 -> Add1/1
  Gain/1 -> dataOut/1

== system benchlink/HDL_64QAM/HDLRxIPCore/QAM Rx HDL/Enabled AGC1/Energy Detector/Variance Estimate2/Moving_Average ==
  dataIn : Inport
  Add : Sum  Inputs=-+  AccumDataTypeStr=fixdt(1,32,18)
  Add1 : Sum  OutDataTypeStr=fixdt(1,32,18)  AccumDataTypeStr=fixdt(1,32,18)
  Delay : Delay  DelayLength=qam_params.golayLength*qam_params.Upsampling*3
  Delay10 : Delay  DelayLength=1  InitialCondition=0  UseCircularBuffer=on
  Delay4 : Delay  DelayLength=1  InitialCondition=0  UseCircularBuffer=on
  Gain : Gain  Gain=1/(qam_params.longTrainingChipLength/4)  OutDataTypeStr=fixdt(1,32,23)
  dataOut : Outport  VectorParamsAs1DForOutWhenUnconnected=off
  wires:
  Add/1 -> Delay10/1
  dataIn/1 -> Delay/1, Add/2
  Delay10/1 -> Add1/2
  Add1/1 -> Gain/1, Delay4/1
  Delay/1 -> Add/1
  Delay4/1 -> Add1/1
  Gain/1 -> dataOut/1

== system benchlink/HDL_64QAM/HDLRxIPCore/QAM Rx HDL/Enabled AGC2/Energy Detector/Variance Estimate/Moving_Average ==
  dataIn : Inport
  Add : Sum  Inputs=-+  AccumDataTypeStr=fixdt(1,32,18)
  Add1 : Sum  OutDataTypeStr=fixdt(1,32,18)  AccumDataTypeStr=fixdt(1,32,18)
  Delay : Delay  DelayLength=qam_params.golayLength*qam_params.Upsampling*2
  Delay10 : Delay  DelayLength=1  InitialCondition=0  UseCircularBuffer=on
  Delay4 : Delay  DelayLength=1  InitialCondition=0  UseCircularBuffer=on
  Gain : Gain  Gain=1/(qam_params.longTrainingChipLength/4)  OutDataTypeStr=fixdt(1,32,23)
  dataOut : Outport  VectorParamsAs1DForOutWhenUnconnected=off
  wires:
  Add/1 -> Delay10/1
  dataIn/1 -> Delay/1, Add/2
  Delay10/1 -> Add1/2
  Add1/1 -> Gain/1, Delay4/1
  Delay/1 -> Add/1
  Delay4/1 -> Add1/1
  Gain/1 -> dataOut/1

== system benchlink/HDL_64QAM/HDLRxIPCore/QAM Rx HDL/Enabled AGC2/Energy Detector/Variance Estimate2/Moving_Average ==
  dataIn : Inport
  Add : Sum  Inputs=-+  AccumDataTypeStr=fixdt(1,32,18)
  Add1 : Sum  OutDataTypeStr=fixdt(1,32,18)  AccumDataTypeStr=fixdt(1,32,18)
  Delay : Delay  DelayLength=qam_params.golayLength*qam_params.Upsampling*2
  Delay10 : Delay  DelayLength=1  InitialCondition=0  UseCircularBuffer=on
  Delay4 : Delay  DelayLength=1  InitialCondition=0  UseCircularBuffer=on
  Gain : Gain  Gain=1/(qam_params.longTrainingChipLength/4)  OutDataTypeStr=fixdt(1,32,23)
  dataOut : Outport  VectorParamsAs1DForOutWhenUnconnected=off
  wires:
  Add/1 -> Delay10/1
  dataIn/1 -> Delay/1, Add/2
  Delay10/1 -> Add1/2
  Add1/1 -> Gain/1, Delay4/1
  Delay/1 -> Add/1
  Delay4/1 -> Add1/1
  Gain/1 -> dataOut/1

== system benchlink/HDL_64QAM/HDLRxIPCore/QAM Rx HDL/MF Filtering and Despreading/BER/Symbol Accum1/Enabled Wire ==
  In1 : Inport
  Enable : EnablePort
  Out1 : Outport  InitialOutput=0  VectorParamsAs1DForOutWhenUnconnected=off
  wires:
  In1/1 -> Out1/1

== system benchlink/HDL_64QAM/HDLRxIPCore/QAM Rx HDL/MF Filtering and Despreading/BER/Symbol Accum1/Falling Edge Detector ==
  In1 : Inport
  Compare To Constant7 : simulink/Logic and Bit Operations/Compare To Constant  relop===  const=-1  OutDataTypeStr=boolean
  Data Type Conversion : DataTypeConversion  OutDataTypeStr=fixdt(1,2,0)  SaturateOnIntegerOverflow=off  RndMeth=Floor
  Data Type Conversion1 : DataTypeConversion  OutDataTypeStr=fixdt(1,2,0)  SaturateOnIntegerOverflow=off  RndMeth=Floor
  Data Type Conversion2 : DataTypeConversion  OutDataTypeStr=fixdt(1,2,0)  SaturateOnIntegerOverflow=off  RndMeth=Floor
  Delay1 : Delay  DelayLength=1  InitialCondition=0
  Subtract1 : Sum  Inputs=-+
  Out1 : Outport  VectorParamsAs1DForOutWhenUnconnected=off
  wires:
  In1/1 -> Data Type Conversion1/1, Delay1/1
  Delay1/1 -> Data Type Conversion/1
  Subtract1/1 -> Data Type Conversion2/1
  Data Type Conversion/1 -> Subtract1/1
  Data Type Conversion1/1 -> Subtract1/2
  Data Type Conversion2/1 -> Compare To Constant7/1
  Compare To Constant7/1 -> Out1/1

== system benchlink/HDL_64QAM/HDLRxIPCore/QAM Rx HDL/MF Filtering and Despreading/SymEVM/Symbol Accum/Enabled Wire ==
  In1 : Inport
  Enable : EnablePort
  Out1 : Outport  InitialOutput=0  VectorParamsAs1DForOutWhenUnconnected=off
  wires:
  In1/1 -> Out1/1

== system benchlink/HDL_64QAM/HDLRxIPCore/QAM Rx HDL/MF Filtering and Despreading/SymEVM/Symbol Accum/Falling Edge Detector ==
  In1 : Inport
  Compare To Constant7 : simulink/Logic and Bit Operations/Compare To Constant  relop===  const=-1  OutDataTypeStr=boolean
  Data Type Conversion : DataTypeConversion  OutDataTypeStr=fixdt(1,2,0)  SaturateOnIntegerOverflow=off  RndMeth=Floor
  Data Type Conversion1 : DataTypeConversion  OutDataTypeStr=fixdt(1,2,0)  SaturateOnIntegerOverflow=off  RndMeth=Floor
  Data Type Conversion2 : DataTypeConversion  OutDataTypeStr=fixdt(1,2,0)  SaturateOnIntegerOverflow=off  RndMeth=Floor
  Delay1 : Delay  DelayLength=1  InitialCondition=0
  Subtract1 : Sum  Inputs=-+
  Out1 : Outport  VectorParamsAs1DForOutWhenUnconnected=off
  wires:
  In1/1 -> Data Type Conversion1/1, Delay1/1
  Delay1/1 -> Data Type Conversion/1
  Subtract1/1 -> Data Type Conversion2/1
  Data Type Conversion/1 -> Subtract1/1
  Data Type Conversion1/1 -> Subtract1/2
  Data Type Conversion2/1 -> Compare To Constant7/1
  Compare To Constant7/1 -> Out1/1

== matlab function benchlink/HDL_64QAM/HDLTxIPCore/QAMTxHDL/Async FIFO/acessControl ==
  data: pop_data output; count input; access_per_burst input; access_lut_position output; is_access output
function [pop_data, access_lut_position, is_access] = accessControl(count, access_per_burst)
%#codegen
% Combines logic for window checking:
%   pop_data:      1 if (count+1) is NOT in a 0-15 window, else 0.
%   access_lut_position: Position (0-15) if count is in window, else 0.
%   is_access:            1 if count IS in a 0-15 window, else 0.
% Assumes count is uint8, num_blocks is power of 2 dividing 256. Outputs uint8.

    coder.allowpcode('plain');

    % --- Constants and Type Casting ---
    total_range_size = uint16(256);
    window_size      = uint16(16);
    access_per_burst_u16   = uint16(access_per_burst);
    count_u16        = uint16(count);

    % --- Core Calculations ---
    block_spacing = idivide(total_range_size, access_per_burst_u16, 'floor'); % uint16

    % Current position
    position_in_block = mod(count_u16, block_spacing); % uint16

    % Next position (handles wrap-around)
    next_count_u16 = count_u16 + 1;
    next_position_in_block = mod(next_count_u16, block_spacing); % uint16

    % --- Determine Outputs ---

    % Output 1: is_in (based on current position)
    if position_in_block < window_size
        is_access = boolean(1);
        access_lut_position = uint8(position_in_block); % Output 2a
    else
        is_access = boolean(0);
        access_lut_position = uint8(0);             % Output 2b
    end

    % Output 3: predict_inv (based on next position)
    if next_position_in_block < window_size
        pop_data = boolean(0);
    else
        pop_data = boolean(1);
    end

end

== matlab function benchlink/HDL_64QAM/HDLRxIPCore/QAM Rx HDL/DA CFC_Avg/Frequency Offset Estimation/KeepMax1 ==
  data: in input; out output; qam_params parameter
function out  = keepMax(in, qam_params)

persistent x counter frameLen

if isempty(x)
    x = fi(0,1,64,46);
    counter    = uint16(0);
    frameLen = uint16((qam_params.packetSymLengthBig*qam_params.spreadingFactor+...
        qam_params.preambleSymLength)*qam_params.Upsampling);
    %frameLen = uint16((qam_params.packetSymLength*qam_params.spreadingFactor+...
    %    qam_params.preambleSymLength)*qam_params.Upsampling);
end

if (counter ~= 0)
    x = max(x,in);
    out = fi(x,1,64,46);
    counter = counter - 1;
else
    if (x > 5*in)
         out = fi(x,1,64,46);
         counter = frameLen;
    else
        x = fi(in,1,64,46);
        out = fi(x,1,64,46);
        counter = frameLen;
    end
end

== matlab function benchlink/HDL_64QAM/HDLRxIPCore/QAM Rx HDL/burstControl ==
  data: switchControl output; packetsPerBurst input; packetSymLength output
function [switchControl,packetSymLength]  = burstControl(packetsPerBurst)
    %#codegen    % Output logic based on the control input value
    if packetsPerBurst == 8 
        switchControl = uint16(2);
        packetSymLength = uint16(2048);
    elseif packetsPerBurst == 4 
        switchControl = uint16(1);
        packetSymLength = uint16(1024);
    else
        switchControl = uint16(2);
        packetSymLength = uint16(2048);
    end
end

== matlab function benchlink/HDL_64QAM/HDLRxIPCore/QAM Rx HDL/DA CFC_Avg/Frequency Offset Estimation/KeepMax ==
  data: in input; out output; qam_params parameter
function out  = keepMax(in, qam_params)

persistent x counter frameLen

if isempty(x)
    x = fi(0,1,64,46);
    counter    = uint16(0);
    frameLen = uint16((qam_params.packetSymLength*qam_params.spreadingFactor+...
        qam_params.preambleSymLength)*qam_params.Upsampling);
    %frameLen = uint16((qam_params.packetSymLength*qam_params.spreadingFactor+...
    %    qam_params.preambleSymLength)*qam_params.Upsampling);
end

if (counter ~= 0)
    x = max(x,in);
    out = fi(x,1,64,46);
    counter = counter - 1;
else
    if (x > 5*in)
         out = fi(x,1,64,46);
         counter = frameLen;
    else
        x = fi(in,1,64,46);
        out = fi(x,1,64,46);
        counter = frameLen;
    end
end

== matlab function benchlink/HDL_64QAM/HDLTxIPCore/QAMTxHDL/Async FIFO/payloadControl1 ==
  data: output output; controlInput input
function output  = payloadControl(controlInput)
    %#codegen    % Output logic based on the control input value
    if controlInput <= 15
        output = uint16(1);
    elseif controlInput == 16
        output = uint16(2);
    else
        output = uint16(3);
    end
end

== matlab function benchlink/HDL_64QAM/HDLRxIPCore/QAM Rx HDL/MF Filtering and Despreading/ Integrate and Dump ==
  data: dValid input; validOut output; symbolIn input; sumOut output
function [validOut, sumOut] = intDump(dValid, symbolIn)
%#codegen

persistent sum_so_far counter

sumOut = fi(complex(0,0),1,18,13);
if isempty(sum_so_far)
sum_so_far = fi(complex(0,0),1,18,13);
end
validOut = false;
if isempty(counter)
counter = uint8(0);
end

if dValid
sum_so_far = fi(sum([sum_so_far symbolIn]),1,18,13);
counter = counter + 1;
end

if counter == 8
    sumOut = sum_so_far;
    validOut = true;
    counter = uint8(0);
    sum_so_far = fi(complex(0,0),1,18,13);
end

end
